simulink model "xieboduoji_13fangzhennow"  (R2023a)
settings: Solver=ode4  StartTime=0.0  StopTime=2.2  FixedStep=5e-7  RelTol=1e-3
undefined symbols (not defined in the file or in its folder): magnitude
libraries: simulink x417, spsRMSLib x70, spsCurrentMeasurementLib x32, spsVoltageMeasurementLib x31, powerlib_meascontrol x24, spsFourierLib x21, spsGroundLib x19, spsThreePhasePISectionLineLib x17, spsThreePhaseSeriesRLCBranchLib x14, spsdq0toAlphaBetaZeroLib x13, spsSeriesRLCBranchLib x11, spsUniversalBridgeLib x11
(part 12 of 12)

== matlab function xieboduoji_13fangzhennow/node5/Subsystem2/RMS1/xunidiandao ==
  data: y1 output; u1 input; u2 input; u3 input; u4 input; u5 input; u6 input; y11 output; y2 output; y22 output; y3 output; y33 output; y4 output; y44 output; y5 output; y55 output; y6 output; y66 output; x output
function [y1,y11,y2,y22,y3,y33,y4,y44,y5,y55,y6,y66,x] = Algorithm(u1,u2,u3,u4,u5,u6)

%控制器参数
T=5e-5;
persistent time;
persistent sum1 sum2 sum3 sum4 sum5 sum6;
persistent sum11 sum22 sum33 sum44 sum55 sum66;
persistent a1 a11 a2 a22 a3 a33 a4 a44 a5 a55 a6 a66
dataType = 'double';

%首次赋值
 if isempty(time)
time=20e-5;
sum1=0;sum2=0;sum3=0;sum4=0;sum5=0;sum6=0;
sum11=0;sum22=0;sum33=0;sum44=0;sum55=0;sum66=0;
a1=0;a11=0;a2=0;a22=0;a3=0;a33=0;a4=0;a44=0;a5=0;a55=0;a6=0;a66=0;
 end

 time=time+T;
  
 if (time>=0.9)&&(time<1.0)
     sum1=sum1+u1;sum2=sum2+u2;sum3=sum3+u3;
     sum4=sum4+u4;sum5=sum5+u5;sum6=sum6+u6;
 end
 if time>=1.0
     a1=sum1*0.0005;a2=sum2*0.0005;a3=sum3*0.0005;
     a4=sum4*0.0005;a5=sum5*0.0005;a6=sum6*0.0005;
 end
  if (time>=1.9)&&(time<2.0)
     sum11=sum11+u1;sum22=sum22+u2;sum33=sum33+u3;
     sum44=sum44+u4;sum55=sum55+u5;sum66=sum66+u6;
 end
 if time>=2.0
     a11=sum11*0.0005;a22=sum22*0.0005;a33=sum33*0.0005;
     a44=sum44*0.0005;a55=sum55*0.0005;a66=sum66*0.0005;
 end
 y1=a1;y2=a2;y3=a3;y4=a4;y5=a5;y6=a6;
 y11=a11;y22=a22;y33=a33;y44=a44;y55=a55;y66=a66;x=time+sum1;
end

== matlab function xieboduoji_13fangzhennow/node5/谐波源/Subsystem1/RMS1/xunidiandao ==
  data: y1 output; u1 input; u2 input; u3 input; u4 input; u5 input; u6 input; y11 output; y2 output; y22 output; y3 output; y33 output; y4 output; y44 output; y5 output; y55 output; y6 output; y66 output; x output
function [y1,y11,y2,y22,y3,y33,y4,y44,y5,y55,y6,y66,x] = Algorithm(u1,u2,u3,u4,u5,u6)

%控制器参数
T=5e-5;
persistent time;
persistent sum1 sum2 sum3 sum4 sum5 sum6;
persistent sum11 sum22 sum33 sum44 sum55 sum66;
persistent a1 a11 a2 a22 a3 a33 a4 a44 a5 a55 a6 a66
dataType = 'double';

%首次赋值
 if isempty(time)
time=20e-5;
sum1=0;sum2=0;sum3=0;sum4=0;sum5=0;sum6=0;
sum11=0;sum22=0;sum33=0;sum44=0;sum55=0;sum66=0;
a1=0;a11=0;a2=0;a22=0;a3=0;a33=0;a4=0;a44=0;a5=0;a55=0;a6=0;a66=0;
 end

 time=time+T;
  
 if (time>=0.9)&&(time<1.0)
     sum1=sum1+u1;sum2=sum2+u2;sum3=sum3+u3;
     sum4=sum4+u4;sum5=sum5+u5;sum6=sum6+u6;
 end
 if time>=1.0
     a1=sum1*0.0005;a2=sum2*0.0005;a3=sum3*0.0005;
     a4=sum4*0.0005;a5=sum5*0.0005;a6=sum6*0.0005;
 end
  if (time>=1.9)&&(time<2.0)
     sum11=sum11+u1;sum22=sum22+u2;sum33=sum33+u3;
     sum44=sum44+u4;sum55=sum55+u5;sum66=sum66+u6;
 end
 if time>=2.0
     a11=sum11*0.0005;a22=sum22*0.0005;a33=sum33*0.0005;
     a44=sum44*0.0005;a55=sum55*0.0005;a66=sum66*0.0005;
 end
 y1=a1;y2=a2;y3=a3;y4=a4;y5=a5;y6=a6;
 y11=a11;y22=a22;y33=a33;y44=a44;y55=a55;y66=a66;x=time+sum1;
end

== matlab function xieboduoji_13fangzhennow/node5/谐波源/Subsystem2/RMS1/xunidiandao ==
  data: y1 output; u1 input; u2 input; u3 input; u4 input; u5 input; u6 input; y11 output; y2 output; y22 output; y3 output; y33 output; y4 output; y44 output; y5 output; y55 output; y6 output; y66 output; x output
function [y1,y11,y2,y22,y3,y33,y4,y44,y5,y55,y6,y66,x] = Algorithm(u1,u2,u3,u4,u5,u6)

%控制器参数
T=5e-5;
persistent time;
persistent sum1 sum2 sum3 sum4 sum5 sum6;
persistent sum11 sum22 sum33 sum44 sum55 sum66;
persistent a1 a11 a2 a22 a3 a33 a4 a44 a5 a55 a6 a66
dataType = 'double';

%首次赋值
 if isempty(time)
time=20e-5;
sum1=0;sum2=0;sum3=0;sum4=0;sum5=0;sum6=0;
sum11=0;sum22=0;sum33=0;sum44=0;sum55=0;sum66=0;
a1=0;a11=0;a2=0;a22=0;a3=0;a33=0;a4=0;a44=0;a5=0;a55=0;a6=0;a66=0;
 end

 time=time+T;
  
 if (time>=0.9)&&(time<1.0)
     sum1=sum1+u1;sum2=sum2+u2;sum3=sum3+u3;
     sum4=sum4+u4;sum5=sum5+u5;sum6=sum6+u6;
 end
 if time>=1.0
     a1=sum1*0.0005;a2=sum2*0.0005;a3=sum3*0.0005;
     a4=sum4*0.0005;a5=sum5*0.0005;a6=sum6*0.0005;
 end
  if (time>=1.9)&&(time<2.0)
     sum11=sum11+u1;sum22=sum22+u2;sum33=sum33+u3;
     sum44=sum44+u4;sum55=sum55+u5;sum66=sum66+u6;
 end
 if time>=2.0
     a11=sum11*0.0005;a22=sum22*0.0005;a33=sum33*0.0005;
     a44=sum44*0.0005;a55=sum55*0.0005;a66=sum66*0.0005;
 end
 y1=a1;y2=a2;y3=a3;y4=a4;y5=a5;y6=a6;
 y11=a11;y22=a22;y33=a33;y44=a44;y55=a55;y66=a66;x=time+sum1;
end

== matlab function xieboduoji_13fangzhennow/node3/PV15kW2/Subsystem9/integral /Embedded MATLAB Function ==
  data: er input; w output
function w  = Algorithm(er)

%控制器参数
Ts=10e-5;%控制周期，原始0.3-6
Kp=0.3;Ki0=8;n=35;
persistent n_sum dcbaohe Ki;
dataType = 'double';

%首次赋值
if isempty(n_sum)
    n_sum=0;dcbaohe=0;Ki=Ki0;
end
 
     n_sum=Ki*Ts*(er)+n_sum;
     outn=Kp*(er)+n_sum;
     if(outn>n)
     outn=n;Ki=0;dcbaohe=1;
     end
     if(outn<-n)
     outn=-n;Ki=0;dcbaohe=1;
     end
     if(dcbaohe==0)
         Ki=Ki0;
     end
     dcbaohe=0;
     
  w=outn; 
end

== matlab function xieboduoji_13fangzhennow/node10/Subsystem1/RMS1/xunidiandao ==
  data: y1 output; u1 input; u2 input; u3 input; u4 input; u5 input; u6 input; y11 output; y2 output; y22 output; y3 output; y33 output; y4 output; y44 output; y5 output; y55 output; y6 output; y66 output; x output
function [y1,y11,y2,y22,y3,y33,y4,y44,y5,y55,y6,y66,x] = Algorithm(u1,u2,u3,u4,u5,u6)

%控制器参数
T=5e-5;
persistent time;
persistent sum1 sum2 sum3 sum4 sum5 sum6;
persistent sum11 sum22 sum33 sum44 sum55 sum66;
persistent a1 a11 a2 a22 a3 a33 a4 a44 a5 a55 a6 a66
dataType = 'double';

%首次赋值
 if isempty(time)
time=20e-5;
sum1=0;sum2=0;sum3=0;sum4=0;sum5=0;sum6=0;
sum11=0;sum22=0;sum33=0;sum44=0;sum55=0;sum66=0;
a1=0;a11=0;a2=0;a22=0;a3=0;a33=0;a4=0;a44=0;a5=0;a55=0;a6=0;a66=0;
 end

 time=time+T;
  
 if (time>=0.9)&&(time<1.0)
     sum1=sum1+u1;sum2=sum2+u2;sum3=sum3+u3;
     sum4=sum4+u4;sum5=sum5+u5;sum6=sum6+u6;
 end
 if time>=1.0
     a1=sum1*0.0005;a2=sum2*0.0005;a3=sum3*0.0005;
     a4=sum4*0.0005;a5=sum5*0.0005;a6=sum6*0.0005;
 end
  if (time>=1.9)&&(time<2.0)
     sum11=sum11+u1;sum22=sum22+u2;sum33=sum33+u3;
     sum44=sum44+u4;sum55=sum55+u5;sum66=sum66+u6;
 end
 if time>=2.0
     a11=sum11*0.0005;a22=sum22*0.0005;a33=sum33*0.0005;
     a44=sum44*0.0005;a55=sum55*0.0005;a66=sum66*0.0005;
 end
 y1=a1;y2=a2;y3=a3;y4=a4;y5=a5;y6=a6;
 y11=a11;y22=a22;y33=a33;y44=a44;y55=a55;y66=a66;x=time+sum1;
end

== matlab function xieboduoji_13fangzhennow/node10/Subsystem2/RMS1/xunidiandao ==
  data: y1 output; u1 input; u2 input; u3 input; u4 input; u5 input; u6 input; y11 output; y2 output; y22 output; y3 output; y33 output; y4 output; y44 output; y5 output; y55 output; y6 output; y66 output; x output
function [y1,y11,y2,y22,y3,y33,y4,y44,y5,y55,y6,y66,x] = Algorithm(u1,u2,u3,u4,u5,u6)

%控制器参数
T=5e-5;
persistent time;
persistent sum1 sum2 sum3 sum4 sum5 sum6;
persistent sum11 sum22 sum33 sum44 sum55 sum66;
persistent a1 a11 a2 a22 a3 a33 a4 a44 a5 a55 a6 a66
dataType = 'double';

%首次赋值
 if isempty(time)
time=20e-5;
sum1=0;sum2=0;sum3=0;sum4=0;sum5=0;sum6=0;
sum11=0;sum22=0;sum33=0;sum44=0;sum55=0;sum66=0;
a1=0;a11=0;a2=0;a22=0;a3=0;a33=0;a4=0;a44=0;a5=0;a55=0;a6=0;a66=0;
 end

 time=time+T;
  
 if (time>=0.9)&&(time<1.0)
     sum1=sum1+u1;sum2=sum2+u2;sum3=sum3+u3;
     sum4=sum4+u4;sum5=sum5+u5;sum6=sum6+u6;
 end
 if time>=1.0
     a1=sum1*0.0005;a2=sum2*0.0005;a3=sum3*0.0005;
     a4=sum4*0.0005;a5=sum5*0.0005;a6=sum6*0.0005;
 end
  if (time>=1.9)&&(time<2.0)
     sum11=sum11+u1;sum22=sum22+u2;sum33=sum33+u3;
     sum44=sum44+u4;sum55=sum55+u5;sum66=sum66+u6;
 end
 if time>=2.0
     a11=sum11*0.0005;a22=sum22*0.0005;a33=sum33*0.0005;
     a44=sum44*0.0005;a55=sum55*0.0005;a66=sum66*0.0005;
 end
 y1=a1;y2=a2;y3=a3;y4=a4;y5=a5;y6=a6;
 y11=a11;y22=a22;y33=a33;y44=a44;y55=a55;y66=a66;x=time+sum1;
end

== matlab function xieboduoji_13fangzhennow/node10/谐波源/Subsystem1/RMS1/xunidiandao ==
  data: y1 output; u1 input; u2 input; u3 input; u4 input; u5 input; u6 input; y11 output; y2 output; y22 output; y3 output; y33 output; y4 output; y44 output; y5 output; y55 output; y6 output; y66 output; x output
function [y1,y11,y2,y22,y3,y33,y4,y44,y5,y55,y6,y66,x] = Algorithm(u1,u2,u3,u4,u5,u6)

%控制器参数
T=5e-5;
persistent time;
persistent sum1 sum2 sum3 sum4 sum5 sum6;
persistent sum11 sum22 sum33 sum44 sum55 sum66;
persistent a1 a11 a2 a22 a3 a33 a4 a44 a5 a55 a6 a66
dataType = 'double';

%首次赋值
 if isempty(time)
time=20e-5;
sum1=0;sum2=0;sum3=0;sum4=0;sum5=0;sum6=0;
sum11=0;sum22=0;sum33=0;sum44=0;sum55=0;sum66=0;
a1=0;a11=0;a2=0;a22=0;a3=0;a33=0;a4=0;a44=0;a5=0;a55=0;a6=0;a66=0;
 end

 time=time+T;
  
 if (time>=0.9)&&(time<1.0)
     sum1=sum1+u1;sum2=sum2+u2;sum3=sum3+u3;
     sum4=sum4+u4;sum5=sum5+u5;sum6=sum6+u6;
 end
 if time>=1.0
     a1=sum1*0.0005;a2=sum2*0.0005;a3=sum3*0.0005;
     a4=sum4*0.0005;a5=sum5*0.0005;a6=sum6*0.0005;
 end
  if (time>=1.9)&&(time<2.0)
     sum11=sum11+u1;sum22=sum22+u2;sum33=sum33+u3;
     sum44=sum44+u4;sum55=sum55+u5;sum66=sum66+u6;
 end
 if time>=2.0
     a11=sum11*0.0005;a22=sum22*0.0005;a33=sum33*0.0005;
     a44=sum44*0.0005;a55=sum55*0.0005;a66=sum66*0.0005;
 end
 y1=a1;y2=a2;y3=a3;y4=a4;y5=a5;y6=a6;
 y11=a11;y22=a22;y33=a33;y44=a44;y55=a55;y66=a66;x=time+sum1;
end

== matlab function xieboduoji_13fangzhennow/node3/PV15kW2/谐波检测/Subsystem2/RMS1/Embedded MATLAB Function ==
  data: ki output; u input
function ki   = Algorithm(u)

%控制器参数
T=5e-5;%控制周期
lim=3;
persistent um k time;
dataType = 'double';

%首次赋值
 if isempty(k)
 um=0;k=1;time=5e-5;
 end
  um=u;
  time=time+T;
  k=lim/um;
%      if k>1
%          k=1;
%      end
 if time<1
     k=1;
 end
 y=um;ki=k;
end

== matlab function xieboduoji_13fangzhennow/node10/谐波源/Subsystem2/RMS1/xunidiandao ==
  data: y1 output; u1 input; u2 input; u3 input; u4 input; u5 input; u6 input; y11 output; y2 output; y22 output; y3 output; y33 output; y4 output; y44 output; y5 output; y55 output; y6 output; y66 output; x output
function [y1,y11,y2,y22,y3,y33,y4,y44,y5,y55,y6,y66,x] = Algorithm(u1,u2,u3,u4,u5,u6)

%控制器参数
T=5e-5;
persistent time;
persistent sum1 sum2 sum3 sum4 sum5 sum6;
persistent sum11 sum22 sum33 sum44 sum55 sum66;
persistent a1 a11 a2 a22 a3 a33 a4 a44 a5 a55 a6 a66
dataType = 'double';

%首次赋值
 if isempty(time)
time=20e-5;
sum1=0;sum2=0;sum3=0;sum4=0;sum5=0;sum6=0;
sum11=0;sum22=0;sum33=0;sum44=0;sum55=0;sum66=0;
a1=0;a11=0;a2=0;a22=0;a3=0;a33=0;a4=0;a44=0;a5=0;a55=0;a6=0;a66=0;
 end

 time=time+T;
  
 if (time>=0.9)&&(time<1.0)
     sum1=sum1+u1;sum2=sum2+u2;sum3=sum3+u3;
     sum4=sum4+u4;sum5=sum5+u5;sum6=sum6+u6;
 end
 if time>=1.0
     a1=sum1*0.0005;a2=sum2*0.0005;a3=sum3*0.0005;
     a4=sum4*0.0005;a5=sum5*0.0005;a6=sum6*0.0005;
 end
  if (time>=1.9)&&(time<2.0)
     sum11=sum11+u1;sum22=sum22+u2;sum33=sum33+u3;
     sum44=sum44+u4;sum55=sum55+u5;sum66=sum66+u6;
 end
 if time>=2.0
     a11=sum11*0.0005;a22=sum22*0.0005;a33=sum33*0.0005;
     a44=sum44*0.0005;a55=sum55*0.0005;a66=sum66*0.0005;
 end
 y1=a1;y2=a2;y3=a3;y4=a4;y5=a5;y6=a6;
 y11=a11;y22=a22;y33=a33;y44=a44;y55=a55;y66=a66;x=time+sum1;
end

== matlab function xieboduoji_13fangzhennow/node8/Subsystem1/RMS1/xunidiandao ==
  data: y1 output; u1 input; u2 input; u3 input; u4 input; u5 input; u6 input; y11 output; y2 output; y22 output; y3 output; y33 output; y4 output; y44 output; y5 output; y55 output; y6 output; y66 output; x output
function [y1,y11,y2,y22,y3,y33,y4,y44,y5,y55,y6,y66,x] = Algorithm(u1,u2,u3,u4,u5,u6)

%控制器参数
T=5e-5;
persistent time;
persistent sum1 sum2 sum3 sum4 sum5 sum6;
persistent sum11 sum22 sum33 sum44 sum55 sum66;
persistent a1 a11 a2 a22 a3 a33 a4 a44 a5 a55 a6 a66
dataType = 'double';

%首次赋值
 if isempty(time)
time=20e-5;
sum1=0;sum2=0;sum3=0;sum4=0;sum5=0;sum6=0;
sum11=0;sum22=0;sum33=0;sum44=0;sum55=0;sum66=0;
a1=0;a11=0;a2=0;a22=0;a3=0;a33=0;a4=0;a44=0;a5=0;a55=0;a6=0;a66=0;
 end

 time=time+T;
  
 if (time>=0.9)&&(time<1.0)
     sum1=sum1+u1;sum2=sum2+u2;sum3=sum3+u3;
     sum4=sum4+u4;sum5=sum5+u5;sum6=sum6+u6;
 end
 if time>=1.0
     a1=sum1*0.0005;a2=sum2*0.0005;a3=sum3*0.0005;
     a4=sum4*0.0005;a5=sum5*0.0005;a6=sum6*0.0005;
 end
  if (time>=1.9)&&(time<2.0)
     sum11=sum11+u1;sum22=sum22+u2;sum33=sum33+u3;
     sum44=sum44+u4;sum55=sum55+u5;sum66=sum66+u6;
 end
 if time>=2.0
     a11=sum11*0.0005;a22=sum22*0.0005;a33=sum33*0.0005;
     a44=sum44*0.0005;a55=sum55*0.0005;a66=sum66*0.0005;
 end
 y1=a1;y2=a2;y3=a3;y4=a4;y5=a5;y6=a6;
 y11=a11;y22=a22;y33=a33;y44=a44;y55=a55;y66=a66;x=time+sum1;
end

== matlab function xieboduoji_13fangzhennow/node8/Subsystem2/RMS1/xunidiandao ==
  data: y1 output; u1 input; u2 input; u3 input; u4 input; u5 input; u6 input; y11 output; y2 output; y22 output; y3 output; y33 output; y4 output; y44 output; y5 output; y55 output; y6 output; y66 output; x output
function [y1,y11,y2,y22,y3,y33,y4,y44,y5,y55,y6,y66,x] = Algorithm(u1,u2,u3,u4,u5,u6)

%控制器参数
T=5e-5;
persistent time;
persistent sum1 sum2 sum3 sum4 sum5 sum6;
persistent sum11 sum22 sum33 sum44 sum55 sum66;
persistent a1 a11 a2 a22 a3 a33 a4 a44 a5 a55 a6 a66
dataType = 'double';

%首次赋值
 if isempty(time)
time=20e-5;
sum1=0;sum2=0;sum3=0;sum4=0;sum5=0;sum6=0;
sum11=0;sum22=0;sum33=0;sum44=0;sum55=0;sum66=0;
a1=0;a11=0;a2=0;a22=0;a3=0;a33=0;a4=0;a44=0;a5=0;a55=0;a6=0;a66=0;
 end

 time=time+T;
  
 if (time>=0.9)&&(time<1.0)
     sum1=sum1+u1;sum2=sum2+u2;sum3=sum3+u3;
     sum4=sum4+u4;sum5=sum5+u5;sum6=sum6+u6;
 end
 if time>=1.0
     a1=sum1*0.0005;a2=sum2*0.0005;a3=sum3*0.0005;
     a4=sum4*0.0005;a5=sum5*0.0005;a6=sum6*0.0005;
 end
  if (time>=1.9)&&(time<2.0)
     sum11=sum11+u1;sum22=sum22+u2;sum33=sum33+u3;
     sum44=sum44+u4;sum55=sum55+u5;sum66=sum66+u6;
 end
 if time>=2.0
     a11=sum11*0.0005;a22=sum22*0.0005;a33=sum33*0.0005;
     a44=sum44*0.0005;a55=sum55*0.0005;a66=sum66*0.0005;
 end
 y1=a1;y2=a2;y3=a3;y4=a4;y5=a5;y6=a6;
 y11=a11;y22=a22;y33=a33;y44=a44;y55=a55;y66=a66;x=time+sum1;
end

== matlab function xieboduoji_13fangzhennow/node3/PV15kW2/谐波检测/Subsystem3/RMS1/Embedded MATLAB Function ==
  data: ki output; u input; y output
function [ki,y]  = Algorithm(u)

%控制器参数
T=5e-5;%控制周期
persistent j1 um us k time;
dataType = 'double';

%首次赋值
 if isempty(j1)
 j1=400;um=0;us=0;k=1;time=0;
 end
 
 time=time+T;
 u2=u*u;
    if(j1>0)
     us=u2+us;j1=j1-1;
    end
    if(j1==0)
     um=us*0.0025;j1=400;us=0;
    end
  if sqrt(um)>3
     k=3/sqrt(um);
  end
  if sqrt(um)<3
     k=sqrt(um)/3;
     if k>1
         k=1;
     end
  end
 if time<1
     k=1;
 end
 y=sqrt(um);ki=k;
% y=um;
end

== matlab function xieboduoji_13fangzhennow/node8/谐波源/Subsystem1/RMS1/xunidiandao ==
  data: y1 output; u1 input; u2 input; u3 input; u4 input; u5 input; u6 input; y11 output; y2 output; y22 output; y3 output; y33 output; y4 output; y44 output; y5 output; y55 output; y6 output; y66 output; x output
function [y1,y11,y2,y22,y3,y33,y4,y44,y5,y55,y6,y66,x] = Algorithm(u1,u2,u3,u4,u5,u6)

%控制器参数
T=5e-5;
persistent time;
persistent sum1 sum2 sum3 sum4 sum5 sum6;
persistent sum11 sum22 sum33 sum44 sum55 sum66;
persistent a1 a11 a2 a22 a3 a33 a4 a44 a5 a55 a6 a66
dataType = 'double';

%首次赋值
 if isempty(time)
time=20e-5;
sum1=0;sum2=0;sum3=0;sum4=0;sum5=0;sum6=0;
sum11=0;sum22=0;sum33=0;sum44=0;sum55=0;sum66=0;
a1=0;a11=0;a2=0;a22=0;a3=0;a33=0;a4=0;a44=0;a5=0;a55=0;a6=0;a66=0;
 end

 time=time+T;
  
 if (time>=0.9)&&(time<1.0)
     sum1=sum1+u1;sum2=sum2+u2;sum3=sum3+u3;
     sum4=sum4+u4;sum5=sum5+u5;sum6=sum6+u6;
 end
 if time>=1.0
     a1=sum1*0.0005;a2=sum2*0.0005;a3=sum3*0.0005;
     a4=sum4*0.0005;a5=sum5*0.0005;a6=sum6*0.0005;
 end
  if (time>=1.9)&&(time<2.0)
     sum11=sum11+u1;sum22=sum22+u2;sum33=sum33+u3;
     sum44=sum44+u4;sum55=sum55+u5;sum66=sum66+u6;
 end
 if time>=2.0
     a11=sum11*0.0005;a22=sum22*0.0005;a33=sum33*0.0005;
     a44=sum44*0.0005;a55=sum55*0.0005;a66=sum66*0.0005;
 end
 y1=a1;y2=a2;y3=a3;y4=a4;y5=a5;y6=a6;
 y11=a11;y22=a22;y33=a33;y44=a44;y55=a55;y66=a66;x=time+sum1;
end

== matlab function xieboduoji_13fangzhennow/node8/谐波源/Subsystem2/RMS1/xunidiandao ==
  data: y1 output; u1 input; u2 input; u3 input; u4 input; u5 input; u6 input; y11 output; y2 output; y22 output; y3 output; y33 output; y4 output; y44 output; y5 output; y55 output; y6 output; y66 output; x output
function [y1,y11,y2,y22,y3,y33,y4,y44,y5,y55,y6,y66,x] = Algorithm(u1,u2,u3,u4,u5,u6)

%控制器参数
T=5e-5;
persistent time;
persistent sum1 sum2 sum3 sum4 sum5 sum6;
persistent sum11 sum22 sum33 sum44 sum55 sum66;
persistent a1 a11 a2 a22 a3 a33 a4 a44 a5 a55 a6 a66
dataType = 'double';

%首次赋值
 if isempty(time)
time=20e-5;
sum1=0;sum2=0;sum3=0;sum4=0;sum5=0;sum6=0;
sum11=0;sum22=0;sum33=0;sum44=0;sum55=0;sum66=0;
a1=0;a11=0;a2=0;a22=0;a3=0;a33=0;a4=0;a44=0;a5=0;a55=0;a6=0;a66=0;
 end

 time=time+T;
  
 if (time>=0.9)&&(time<1.0)
     sum1=sum1+u1;sum2=sum2+u2;sum3=sum3+u3;
     sum4=sum4+u4;sum5=sum5+u5;sum6=sum6+u6;
 end
 if time>=1.0
     a1=sum1*0.0005;a2=sum2*0.0005;a3=sum3*0.0005;
     a4=sum4*0.0005;a5=sum5*0.0005;a6=sum6*0.0005;
 end
  if (time>=1.9)&&(time<2.0)
     sum11=sum11+u1;sum22=sum22+u2;sum33=sum33+u3;
     sum44=sum44+u4;sum55=sum55+u5;sum66=sum66+u6;
 end
 if time>=2.0
     a11=sum11*0.0005;a22=sum22*0.0005;a33=sum33*0.0005;
     a44=sum44*0.0005;a55=sum55*0.0005;a66=sum66*0.0005;
 end
 y1=a1;y2=a2;y3=a3;y4=a4;y5=a5;y6=a6;
 y11=a11;y22=a22;y33=a33;y44=a44;y55=a55;y66=a66;x=time+sum1;
end

== matlab function xieboduoji_13fangzhennow/node14/Subsystem1/RMS1/xunidiandao ==
  data: y1 output; u1 input; u2 input; u3 input; u4 input; u5 input; u6 input; y11 output; y2 output; y22 output; y3 output; y33 output; y4 output; y44 output; y5 output; y55 output; y6 output; y66 output; x output
function [y1,y11,y2,y22,y3,y33,y4,y44,y5,y55,y6,y66,x] = Algorithm(u1,u2,u3,u4,u5,u6)

%控制器参数
T=5e-5;
persistent time;
persistent sum1 sum2 sum3 sum4 sum5 sum6;
persistent sum11 sum22 sum33 sum44 sum55 sum66;
persistent a1 a11 a2 a22 a3 a33 a4 a44 a5 a55 a6 a66
dataType = 'double';

%首次赋值
 if isempty(time)
time=20e-5;
sum1=0;sum2=0;sum3=0;sum4=0;sum5=0;sum6=0;
sum11=0;sum22=0;sum33=0;sum44=0;sum55=0;sum66=0;
a1=0;a11=0;a2=0;a22=0;a3=0;a33=0;a4=0;a44=0;a5=0;a55=0;a6=0;a66=0;
 end

 time=time+T;
  
 if (time>=0.9)&&(time<1.0)
     sum1=sum1+u1;sum2=sum2+u2;sum3=sum3+u3;
     sum4=sum4+u4;sum5=sum5+u5;sum6=sum6+u6;
 end
 if time>=1.0
     a1=sum1*0.0005;a2=sum2*0.0005;a3=sum3*0.0005;
     a4=sum4*0.0005;a5=sum5*0.0005;a6=sum6*0.0005;
 end
  if (time>=1.9)&&(time<2.0)
     sum11=sum11+u1;sum22=sum22+u2;sum33=sum33+u3;
     sum44=sum44+u4;sum55=sum55+u5;sum66=sum66+u6;
 end
 if time>=2.0
     a11=sum11*0.0005;a22=sum22*0.0005;a33=sum33*0.0005;
     a44=sum44*0.0005;a55=sum55*0.0005;a66=sum66*0.0005;
 end
 y1=a1;y2=a2;y3=a3;y4=a4;y5=a5;y6=a6;
 y11=a11;y22=a22;y33=a33;y44=a44;y55=a55;y66=a66;x=time+sum1;
end

== matlab function xieboduoji_13fangzhennow/node3/PV15kW2/谐波检测/DFT6-24A1/Subsystem9/integral /Embedded MATLAB Function ==
  data: er input; w output
function w  = Algorithm(er)

%控制器参数
Ts=5e-5;%控制周期，原始0.3-6
Kp=0;Ki0=5;n=0;
persistent n_sum baohe Ki outn err flg;
dataType = 'double';

%首次赋值
 if isempty(n_sum)
    n_sum=1;baohe=0;Ki=Ki0;outn=1;err=0;flg=0;
 end
     err=er;
     if err<-0.1
         flg=1;
     end
     if (flg==1)&&(err>0)
         flg=0;
     end
 if flg==1 
     n_sum=Ki*Ts*err+n_sum; outn=Kp*err+n_sum;
     if(outn>1)
     outn=1;Ki=0;baohe=1;
     end
     if(outn<0)
     outn=0;Ki=0;baohe=1;
     end
     if(baohe==0)
         Ki=Ki0;
     end
     baohe=0;
 end    
w=outn; 
end

== matlab function xieboduoji_13fangzhennow/node14/Subsystem2/RMS1/xunidiandao ==
  data: y1 output; u1 input; u2 input; u3 input; u4 input; u5 input; u6 input; y11 output; y2 output; y22 output; y3 output; y33 output; y4 output; y44 output; y5 output; y55 output; y6 output; y66 output; x output
function [y1,y11,y2,y22,y3,y33,y4,y44,y5,y55,y6,y66,x] = Algorithm(u1,u2,u3,u4,u5,u6)

%控制器参数
T=5e-5;
persistent time;
persistent sum1 sum2 sum3 sum4 sum5 sum6;
persistent sum11 sum22 sum33 sum44 sum55 sum66;
persistent a1 a11 a2 a22 a3 a33 a4 a44 a5 a55 a6 a66
dataType = 'double';

%首次赋值
 if isempty(time)
time=20e-5;
sum1=0;sum2=0;sum3=0;sum4=0;sum5=0;sum6=0;
sum11=0;sum22=0;sum33=0;sum44=0;sum55=0;sum66=0;
a1=0;a11=0;a2=0;a22=0;a3=0;a33=0;a4=0;a44=0;a5=0;a55=0;a6=0;a66=0;
 end

 time=time+T;
  
 if (time>=0.9)&&(time<1.0)
     sum1=sum1+u1;sum2=sum2+u2;sum3=sum3+u3;
     sum4=sum4+u4;sum5=sum5+u5;sum6=sum6+u6;
 end
 if time>=1.0
     a1=sum1*0.0005;a2=sum2*0.0005;a3=sum3*0.0005;
     a4=sum4*0.0005;a5=sum5*0.0005;a6=sum6*0.0005;
 end
  if (time>=1.9)&&(time<2.0)
     sum11=sum11+u1;sum22=sum22+u2;sum33=sum33+u3;
     sum44=sum44+u4;sum55=sum55+u5;sum66=sum66+u6;
 end
 if time>=2.0
     a11=sum11*0.0005;a22=sum22*0.0005;a33=sum33*0.0005;
     a44=sum44*0.0005;a55=sum55*0.0005;a66=sum66*0.0005;
 end
 y1=a1;y2=a2;y3=a3;y4=a4;y5=a5;y6=a6;
 y11=a11;y22=a22;y33=a33;y44=a44;y55=a55;y66=a66;x=time+sum1;
end

== matlab function xieboduoji_13fangzhennow/node14/谐波源/Subsystem1/RMS1/xunidiandao ==
  data: y1 output; u1 input; u2 input; u3 input; u4 input; u5 input; u6 input; y11 output; y2 output; y22 output; y3 output; y33 output; y4 output; y44 output; y5 output; y55 output; y6 output; y66 output; x output
function [y1,y11,y2,y22,y3,y33,y4,y44,y5,y55,y6,y66,x] = Algorithm(u1,u2,u3,u4,u5,u6)

%控制器参数
T=5e-5;
persistent time;
persistent sum1 sum2 sum3 sum4 sum5 sum6;
persistent sum11 sum22 sum33 sum44 sum55 sum66;
persistent a1 a11 a2 a22 a3 a33 a4 a44 a5 a55 a6 a66
dataType = 'double';

%首次赋值
 if isempty(time)
time=20e-5;
sum1=0;sum2=0;sum3=0;sum4=0;sum5=0;sum6=0;
sum11=0;sum22=0;sum33=0;sum44=0;sum55=0;sum66=0;
a1=0;a11=0;a2=0;a22=0;a3=0;a33=0;a4=0;a44=0;a5=0;a55=0;a6=0;a66=0;
 end

 time=time+T;
  
 if (time>=0.9)&&(time<1.0)
     sum1=sum1+u1;sum2=sum2+u2;sum3=sum3+u3;
     sum4=sum4+u4;sum5=sum5+u5;sum6=sum6+u6;
 end
 if time>=1.0
     a1=sum1*0.0005;a2=sum2*0.0005;a3=sum3*0.0005;
     a4=sum4*0.0005;a5=sum5*0.0005;a6=sum6*0.0005;
 end
  if (time>=1.9)&&(time<2.0)
     sum11=sum11+u1;sum22=sum22+u2;sum33=sum33+u3;
     sum44=sum44+u4;sum55=sum55+u5;sum66=sum66+u6;
 end
 if time>=2.0
     a11=sum11*0.0005;a22=sum22*0.0005;a33=sum33*0.0005;
     a44=sum44*0.0005;a55=sum55*0.0005;a66=sum66*0.0005;
 end
 y1=a1;y2=a2;y3=a3;y4=a4;y5=a5;y6=a6;
 y11=a11;y22=a22;y33=a33;y44=a44;y55=a55;y66=a66;x=time+sum1;
end

== matlab function xieboduoji_13fangzhennow/node14/谐波源/Subsystem2/RMS1/xunidiandao ==
  data: y1 output; u1 input; u2 input; u3 input; u4 input; u5 input; u6 input; y11 output; y2 output; y22 output; y3 output; y33 output; y4 output; y44 output; y5 output; y55 output; y6 output; y66 output; x output
function [y1,y11,y2,y22,y3,y33,y4,y44,y5,y55,y6,y66,x] = Algorithm(u1,u2,u3,u4,u5,u6)

%控制器参数
T=5e-5;
persistent time;
persistent sum1 sum2 sum3 sum4 sum5 sum6;
persistent sum11 sum22 sum33 sum44 sum55 sum66;
persistent a1 a11 a2 a22 a3 a33 a4 a44 a5 a55 a6 a66
dataType = 'double';

%首次赋值
 if isempty(time)
time=20e-5;
sum1=0;sum2=0;sum3=0;sum4=0;sum5=0;sum6=0;
sum11=0;sum22=0;sum33=0;sum44=0;sum55=0;sum66=0;
a1=0;a11=0;a2=0;a22=0;a3=0;a33=0;a4=0;a44=0;a5=0;a55=0;a6=0;a66=0;
 end

 time=time+T;
  
 if (time>=0.9)&&(time<1.0)
     sum1=sum1+u1;sum2=sum2+u2;sum3=sum3+u3;
     sum4=sum4+u4;sum5=sum5+u5;sum6=sum6+u6;
 end
 if time>=1.0
     a1=sum1*0.0005;a2=sum2*0.0005;a3=sum3*0.0005;
     a4=sum4*0.0005;a5=sum5*0.0005;a6=sum6*0.0005;
 end
  if (time>=1.9)&&(time<2.0)
     sum11=sum11+u1;sum22=sum22+u2;sum33=sum33+u3;
     sum44=sum44+u4;sum55=sum55+u5;sum66=sum66+u6;
 end
 if time>=2.0
     a11=sum11*0.0005;a22=sum22*0.0005;a33=sum33*0.0005;
     a44=sum44*0.0005;a55=sum55*0.0005;a66=sum66*0.0005;
 end
 y1=a1;y2=a2;y3=a3;y4=a4;y5=a5;y6=a6;
 y11=a11;y22=a22;y33=a33;y44=a44;y55=a55;y66=a66;x=time+sum1;
end

== matlab function xieboduoji_13fangzhennow/node14/PV15kW3/Subsystem9/integral /Embedded MATLAB Function ==
  data: er input; w output
function w  = Algorithm(er)

%控制器参数
Ts=10e-5;%控制周期，原始0.3-6
Kp=0.3;Ki0=8;n=35;
persistent n_sum dcbaohe Ki;
dataType = 'double';

%首次赋值
if isempty(n_sum)
    n_sum=0;dcbaohe=0;Ki=Ki0;
end
 
     n_sum=Ki*Ts*(er)+n_sum;
     outn=Kp*(er)+n_sum;
     if(outn>n)
     outn=n;Ki=0;dcbaohe=1;
     end
     if(outn<-n)
     outn=-n;Ki=0;dcbaohe=1;
     end
     if(dcbaohe==0)
         Ki=Ki0;
     end
     dcbaohe=0;
     
  w=outn; 
end

== matlab function xieboduoji_13fangzhennow/node12/Subsystem1/RMS1/xunidiandao ==
  data: y1 output; u1 input; u2 input; u3 input; u4 input; u5 input; u6 input; y11 output; y2 output; y22 output; y3 output; y33 output; y4 output; y44 output; y5 output; y55 output; y6 output; y66 output; x output
function [y1,y11,y2,y22,y3,y33,y4,y44,y5,y55,y6,y66,x] = Algorithm(u1,u2,u3,u4,u5,u6)

%控制器参数
T=5e-5;
persistent time;
persistent sum1 sum2 sum3 sum4 sum5 sum6;
persistent sum11 sum22 sum33 sum44 sum55 sum66;
persistent a1 a11 a2 a22 a3 a33 a4 a44 a5 a55 a6 a66
dataType = 'double';

%首次赋值
 if isempty(time)
time=20e-5;
sum1=0;sum2=0;sum3=0;sum4=0;sum5=0;sum6=0;
sum11=0;sum22=0;sum33=0;sum44=0;sum55=0;sum66=0;
a1=0;a11=0;a2=0;a22=0;a3=0;a33=0;a4=0;a44=0;a5=0;a55=0;a6=0;a66=0;
 end

 time=time+T;
  
 if (time>=0.9)&&(time<1.0)
     sum1=sum1+u1;sum2=sum2+u2;sum3=sum3+u3;
     sum4=sum4+u4;sum5=sum5+u5;sum6=sum6+u6;
 end
 if time>=1.0
     a1=sum1*0.0005;a2=sum2*0.0005;a3=sum3*0.0005;
     a4=sum4*0.0005;a5=sum5*0.0005;a6=sum6*0.0005;
 end
  if (time>=1.9)&&(time<2.0)
     sum11=sum11+u1;sum22=sum22+u2;sum33=sum33+u3;
     sum44=sum44+u4;sum55=sum55+u5;sum66=sum66+u6;
 end
 if time>=2.0
     a11=sum11*0.0005;a22=sum22*0.0005;a33=sum33*0.0005;
     a44=sum44*0.0005;a55=sum55*0.0005;a66=sum66*0.0005;
 end
 y1=a1;y2=a2;y3=a3;y4=a4;y5=a5;y6=a6;
 y11=a11;y22=a22;y33=a33;y44=a44;y55=a55;y66=a66;x=time+sum1;
end

== matlab function xieboduoji_13fangzhennow/node12/Subsystem2/RMS1/xunidiandao ==
  data: y1 output; u1 input; u2 input; u3 input; u4 input; u5 input; u6 input; y11 output; y2 output; y22 output; y3 output; y33 output; y4 output; y44 output; y5 output; y55 output; y6 output; y66 output; x output
function [y1,y11,y2,y22,y3,y33,y4,y44,y5,y55,y6,y66,x] = Algorithm(u1,u2,u3,u4,u5,u6)

%控制器参数
T=5e-5;
persistent time;
persistent sum1 sum2 sum3 sum4 sum5 sum6;
persistent sum11 sum22 sum33 sum44 sum55 sum66;
persistent a1 a11 a2 a22 a3 a33 a4 a44 a5 a55 a6 a66
dataType = 'double';

%首次赋值
 if isempty(time)
time=20e-5;
sum1=0;sum2=0;sum3=0;sum4=0;sum5=0;sum6=0;
sum11=0;sum22=0;sum33=0;sum44=0;sum55=0;sum66=0;
a1=0;a11=0;a2=0;a22=0;a3=0;a33=0;a4=0;a44=0;a5=0;a55=0;a6=0;a66=0;
 end

 time=time+T;
  
 if (time>=0.9)&&(time<1.0)
     sum1=sum1+u1;sum2=sum2+u2;sum3=sum3+u3;
     sum4=sum4+u4;sum5=sum5+u5;sum6=sum6+u6;
 end
 if time>=1.0
     a1=sum1*0.0005;a2=sum2*0.0005;a3=sum3*0.0005;
     a4=sum4*0.0005;a5=sum5*0.0005;a6=sum6*0.0005;
 end
  if (time>=1.9)&&(time<2.0)
     sum11=sum11+u1;sum22=sum22+u2;sum33=sum33+u3;
     sum44=sum44+u4;sum55=sum55+u5;sum66=sum66+u6;
 end
 if time>=2.0
     a11=sum11*0.0005;a22=sum22*0.0005;a33=sum33*0.0005;
     a44=sum44*0.0005;a55=sum55*0.0005;a66=sum66*0.0005;
 end
 y1=a1;y2=a2;y3=a3;y4=a4;y5=a5;y6=a6;
 y11=a11;y22=a22;y33=a33;y44=a44;y55=a55;y66=a66;x=time+sum1;
end

== matlab function xieboduoji_13fangzhennow/node12/谐波源1/Subsystem1/RMS1/xunidiandao ==
  data: y1 output; u1 input; u2 input; u3 input; u4 input; u5 input; u6 input; y11 output; y2 output; y22 output; y3 output; y33 output; y4 output; y44 output; y5 output; y55 output; y6 output; y66 output; x output
function [y1,y11,y2,y22,y3,y33,y4,y44,y5,y55,y6,y66,x] = Algorithm(u1,u2,u3,u4,u5,u6)

%控制器参数
T=5e-5;
persistent time;
persistent sum1 sum2 sum3 sum4 sum5 sum6;
persistent sum11 sum22 sum33 sum44 sum55 sum66;
persistent a1 a11 a2 a22 a3 a33 a4 a44 a5 a55 a6 a66
dataType = 'double';

%首次赋值
 if isempty(time)
time=20e-5;
sum1=0;sum2=0;sum3=0;sum4=0;sum5=0;sum6=0;
sum11=0;sum22=0;sum33=0;sum44=0;sum55=0;sum66=0;
a1=0;a11=0;a2=0;a22=0;a3=0;a33=0;a4=0;a44=0;a5=0;a55=0;a6=0;a66=0;
 end

 time=time+T;
  
 if (time>=0.9)&&(time<1.0)
     sum1=sum1+u1;sum2=sum2+u2;sum3=sum3+u3;
     sum4=sum4+u4;sum5=sum5+u5;sum6=sum6+u6;
 end
 if time>=1.0
     a1=sum1*0.0005;a2=sum2*0.0005;a3=sum3*0.0005;
     a4=sum4*0.0005;a5=sum5*0.0005;a6=sum6*0.0005;
 end
  if (time>=1.9)&&(time<2.0)
     sum11=sum11+u1;sum22=sum22+u2;sum33=sum33+u3;
     sum44=sum44+u4;sum55=sum55+u5;sum66=sum66+u6;
 end
 if time>=2.0
     a11=sum11*0.0005;a22=sum22*0.0005;a33=sum33*0.0005;
     a44=sum44*0.0005;a55=sum55*0.0005;a66=sum66*0.0005;
 end
 y1=a1;y2=a2;y3=a3;y4=a4;y5=a5;y6=a6;
 y11=a11;y22=a22;y33=a33;y44=a44;y55=a55;y66=a66;x=time+sum1;
end

== matlab function xieboduoji_13fangzhennow/node14/PV15kW3/改进PLL1/PI/Embedded MATLAB Function ==
  data: Vgq input; w output
function w  = Algorithm(Vgq)

%控制器参数
T=5e-5;%控制周期

Kpllp=0.2;
Kplli=4;

persistent PLLsum;
persistent nsum2;

dataType = 'double';

%首次赋值
if isempty(PLLsum)
    PLLsum=0;
    nsum2=0;
end


w=Kpllp*Vgq+Kplli*(T*Vgq+PLLsum);
PLLsum=T*Vgq+PLLsum;
end

== matlab function xieboduoji_13fangzhennow/node12/谐波源1/Subsystem2/RMS1/xunidiandao ==
  data: y1 output; u1 input; u2 input; u3 input; u4 input; u5 input; u6 input; y11 output; y2 output; y22 output; y3 output; y33 output; y4 output; y44 output; y5 output; y55 output; y6 output; y66 output; x output
function [y1,y11,y2,y22,y3,y33,y4,y44,y5,y55,y6,y66,x] = Algorithm(u1,u2,u3,u4,u5,u6)

%控制器参数
T=5e-5;
persistent time;
persistent sum1 sum2 sum3 sum4 sum5 sum6;
persistent sum11 sum22 sum33 sum44 sum55 sum66;
persistent a1 a11 a2 a22 a3 a33 a4 a44 a5 a55 a6 a66
dataType = 'double';

%首次赋值
 if isempty(time)
time=20e-5;
sum1=0;sum2=0;sum3=0;sum4=0;sum5=0;sum6=0;
sum11=0;sum22=0;sum33=0;sum44=0;sum55=0;sum66=0;
a1=0;a11=0;a2=0;a22=0;a3=0;a33=0;a4=0;a44=0;a5=0;a55=0;a6=0;a66=0;
 end

 time=time+T;
  
 if (time>=0.9)&&(time<1.0)
     sum1=sum1+u1;sum2=sum2+u2;sum3=sum3+u3;
     sum4=sum4+u4;sum5=sum5+u5;sum6=sum6+u6;
 end
 if time>=1.0
     a1=sum1*0.0005;a2=sum2*0.0005;a3=sum3*0.0005;
     a4=sum4*0.0005;a5=sum5*0.0005;a6=sum6*0.0005;
 end
  if (time>=1.9)&&(time<2.0)
     sum11=sum11+u1;sum22=sum22+u2;sum33=sum33+u3;
     sum44=sum44+u4;sum55=sum55+u5;sum66=sum66+u6;
 end
 if time>=2.0
     a11=sum11*0.0005;a22=sum22*0.0005;a33=sum33*0.0005;
     a44=sum44*0.0005;a55=sum55*0.0005;a66=sum66*0.0005;
 end
 y1=a1;y2=a2;y3=a3;y4=a4;y5=a5;y6=a6;
 y11=a11;y22=a22;y33=a33;y44=a44;y55=a55;y66=a66;x=time+sum1;
end

== matlab function xieboduoji_13fangzhennow/node3/PV15kW3/谐波检测/Subsystem/Subsystem2/RMS1/xiebodianliu1 ==
  data: k1 output; u1 input; i1 input; u2 input; i2 input; u3 input; i3 input; u4 input; i4 input; u5 input; i5 input; u6 input; k2 output; k3 output; k4 output; k5 output; k6 output; i6 input; k0 output
function [k1,k2,k3,k4,k5,k6,k0] = Algorithm(u1,i1,u2,i2,u3,i3,u4,i4,u5,i5,u6,i6)

%控制器参数
T=5e-5;
kp=0.01;
persistent lim lim1 im k time;
persistent k11 k22 k33 k44 k55 k66;
persistent flg1 flg2 flg3 flg4 flg5 flg6;
dataType = 'double';

%首次赋值
 if isempty(k)
 lim=5;lim1=5;im=0;k=1;time=5e-5;
 k11=0;k22=0;k33=0;k44=0;k55=0;k66=0;
 flg1=1; flg2=1; flg3=1; flg4=1; flg5=1; flg6=1;
 end
h1=1/0.6464;h2=1/0.7219;h3=1/1;
h4=1/0.9880;h5=1/0.5562;h6=1/0.6416;

im=sqrt(flg1*i1^2+flg2*i2^2+flg3*i3^2+flg4*i4^2+flg5*i5^2+flg6*i6^2);
it=(lim^2-((1-flg1)*h1*i1)^2-((1-flg2)*h2*i2)^2-((1-flg3)*h3*i3)^2-((1-flg4)*h4*i4)^2-((1-flg5)*h5*i5)^2-((1-flg6)*h6*i6)^2);
 if it>=0
 lim1=sqrt(it);
  if im>0
  k=lim1/im;end
 else
 lim1=0;k=0.7;
 end
time=time+T;
 if k>2
 k=2;end
     if k>h1
      k11=h1;flg1=0;
      else
      flg1=1;k11=k;end
     if k>h2
      k22=h2;flg2=0;
      else
      flg2=1;k22=k;end
     if k>h3
      k33=h3;flg3=0;
      else
      flg3=1;k33=k;end
     if k>h4
      k44=h4;flg4=0;
      else
      flg4=1;k44=k;end
     if k>h5
      k55=h5;flg5=0;
      else
      flg5=1;k55=k;end
     if k>h6
      k66=h6;flg6=0;
      else
      flg6=1;k66=k;end

  
 if time<1
     k11=0;k22=0;k33=0;k44=0;k55=0;k66=0;
 end
 if time>=1.4
lim=10.6-time*4.0;lim1=10.6-time*4.0;
    if lim<4
    lim=4;lim1=4;
    end
 end
 
 k1=k11;k2=k22;k3=k33;k4=k44;k5=k55;k6=k66;k0=it;
end

== matlab function xieboduoji_13fangzhennow/node14/PV15kW3/谐波检测/Subsystem2/RMS1/xunidiandao1 ==
  data: k1 output; u1 input; i1 input; u2 input; i2 input; u3 input; i3 input; u4 input; i4 input; u5 input; i5 input; u6 input; k2 output; k3 output; k4 output; k5 output; k6 output; i6 input; k0 output
function [k1,k2,k3,k4,k5,k6,k0] = Algorithm(u1,i1,u2,i2,u3,i3,u4,i4,u5,i5,u6,i6)

%控制器参数
T=5e-5;
kp=0.01;
persistent low lim im k time;
persistent k11 k22 k33 k44 k55 k66;
persistent h6 flg6 sum6 out6 bao6 ki6;
persistent h5 flg5 sum5 out5 bao5 ki5;
dataType = 'double';

%首次赋值
 if isempty(k)
 low=1.244;lim=5;im=0;k=1;time=5e-5;%1.1
 k11=0;k22=0;k33=0;k44=0;k55=0;k66=0;
 h6=1;flg6=1;sum6=1;out6=1;bao6=0;ki6=25;
 h5=1;flg5=1;sum5=1;out5=1;bao5=0;ki5=25;
 end
%    if (flg5==0)&&(flg6==0)
%     if sqrt((i5*out5)^2+(i6*out6)^2)>lim
%          if (flg5>flg6)
%              flg5=1;
%          else
%              flg6=1;
%          end
%     end
%    end  
    if flg5==1
      h5=1;
    else h5=out5/k;end 
    if flg6==1
      h6=1;
    else h6=out6/k;end   
 im=sqrt(i1*i1+i2*i2+i3*i3+i4*i4+(i5*h5)^2+(i6*h6)^2);%
 time=time+T;  
 k=lim/im;
     if k>3
     k=3;end
 k11=k;k22=k;k33=k;k44=k;
     if flg5==1
     k55=k;end
     if flg6==1
     k66=k;end
  
 if time<1
     k11=0;k22=0;k33=0;k44=0;k55=0;k66=0;
 end
 if time>=1
     if time>=1.4
     low=1.02;end%1.02
     if time>=1.7
     low=0.512;end%0.512
  if time>=1.4
lim=10.6-time*4.0;lim1=10.6-time*4.0;
    if lim<4
    lim=4;lim1=4;
    end
  end
  
 er6=u6*1.414-low;er5=u5*1.414-low;
%     if (er5<-0.06)||(er5>0.06)
%          if (er5<-0.06) 
%           if flg5==1
%           sum5=k;out5=k;end
%          flg5=0;end   
%     sum5=ki5*T*er5+sum5;out5=kp*er5+sum5;
%         if flg5==0 
%         k55=out5;end
%      if(out5>k)
%      flg5=1;out5=k;ki5=0;bao5=1;end
%      if(out5<0)
%      out5=0;ki5=0;bao5=1;end
%      if(bao5==0)
%      ki5=25;end
%      bao5=0;
%    end
%     if (er6<-0.06)||(er6>0.06)
%          if (er6<-0.06) 
%            if flg6==1
%            sum6=k;out6=k;end
%          flg6=0;end   
%      sum6=ki6*T*er6+sum6; out6=kp*er6+sum6;
%         if flg6==0 
%         k66=out6;end
%      if(out6>k)
%      flg6=1;out6=k;ki6=0;bao6=1;end
%      if(out6<0)
%      out6=0;ki6=0;bao6=1;end
%      if(bao6==0)
%      ki6=25;end
%      bao6=0;
%     end
 end
 
 k1=k11;k2=k22;k3=k33;k4=k44;k5=k55;k6=k66;k0=flg6;
end

== matlab function xieboduoji_13fangzhennow/node3/PV15kW3/谐波检测/Subsystem2/RMS1/xiebodianliu ==
  data: k1 output; u1 input; i1 input; u2 input; i2 input; u3 input; i3 input; u4 input; i4 input; u5 input; i5 input; u6 input; k2 output; k3 output; k4 output; k5 output; k6 output; i6 input; k0 output
function [k1,k2,k3,k4,k5,k6,k0] = Algorithm(u1,i1,u2,i2,u3,i3,u4,i4,u5,i5,u6,i6)

%控制器参数
T=5e-5;
kp=0.01;
persistent lim im k time;
persistent k11 k22 k33 k44 k55 k66;
persistent flg1 flg2 flg3 flg4 flg5 flg6;
dataType = 'double';

%首次赋值
 if isempty(k)
 lim=6;lim1=6;im=0;k=1;time=5e-5;
 k11=0;k22=0;k33=0;k44=0;k55=0;k66=0;
 flg1=1; flg2=1; flg3=1; flg4=1; flg5=1; flg6=1;
 end
h1=1/0.8;h2=1/0.8;h3=1/0.8;
h4=1/0.8;h5=1/0.8;h6=1/0.8;
%     if flg5==1
%       h5=1;
%     else h5=out5/k;end 
im=sqrt(flg1*i1^2+flg2*i2^2+flg3*i3^2+flg4*i4^2+flg5*i5^2+flg6*i6^2);
lim1=sqrt(lim^2-((1-flg1)*h1*i1)^2-((1-flg2)*h2*i2)^2-((1-flg3)*h3*i3)^2-((1-flg4)*h4*i4)^2-((1-flg5)*h5*i5)^2-((1-flg6)*h6*i6)^2)
time=time+T;  
k=lim1/im;
 if k>5
 k=5;end
     if k>h1
      k11=h1;flg1=0;
      else
      flg1=1;k11=k;end
     if k>h2
      k22=h2;flg2=0;
      else
      flg2=1;k22=k;end
     if k>h3
      k33=h3;flg3=0;
      else
      flg3=1;k33=k;end
     if k>h4
      k44=h4;flg4=0;
      else
      flg4=1;k44=k;end
     if k>h5
      k55=h5;flg5=0;
      else
      flg5=1;k55=k;end
     if k>h6
      k66=h6;flg6=0;
      else
      flg6=1;k66=k;end

  
 if time<1
     k11=0;k22=0;k33=0;k44=0;k55=0;k66=0;
 end
 if time>=1

 end
 
 k1=k11;k2=k22;k3=k33;k4=k44;k5=k55;k6=k66;k0=flg6;
end
